simulink model "B1P3_Torsonal_Model_1_Coupler"  (Simulink 6.5)
settings: Solver=ode23tb  StartTime=0.0  StopTime=0.5  RelTol=1e-3
values from neighbouring files (symbols this model uses):
  B1 = 0    [B1P3_Torsonal_Model_1_Coupler_Constants.m]    (also in B1P6_Torsonal_Model_2_Coupler_Constants.m; Torsonal_Model_Constants.m)
  Bc = 0.01    [B1P3_Torsonal_Model_1_Coupler_Constants.m]    (also in Torsonal_Model_Constants.m)
  BL = 0    [B1P3_Torsonal_Model_1_Coupler_Constants.m]    (also in Torsonal_Model_Constants.m)
  J1 = 0.0033    [B1P3_Torsonal_Model_1_Coupler_Constants.m]    (also in B1P6_Torsonal_Model_2_Coupler_Constants.m = 0.0023; Torsonal_Model_Constants.m = 0.0023)
  JL = 0.0033    [B1P15_Torsonal_Model_From_V_Rizzo_One_Coupler_Constants.m]    (also in B1P3_Torsonal_Model_1_Coupler_Constants.m = 0.0023; RizzoConst.m; Torsonal_Model_Constants.m)
  K = 1000    [B1P3_Torsonal_Model_1_Coupler_Constants.m]    (also in Torsonal_Model_Constants.m = 55)
settings Model: Creator=dml46  LastModifiedBy=dml46

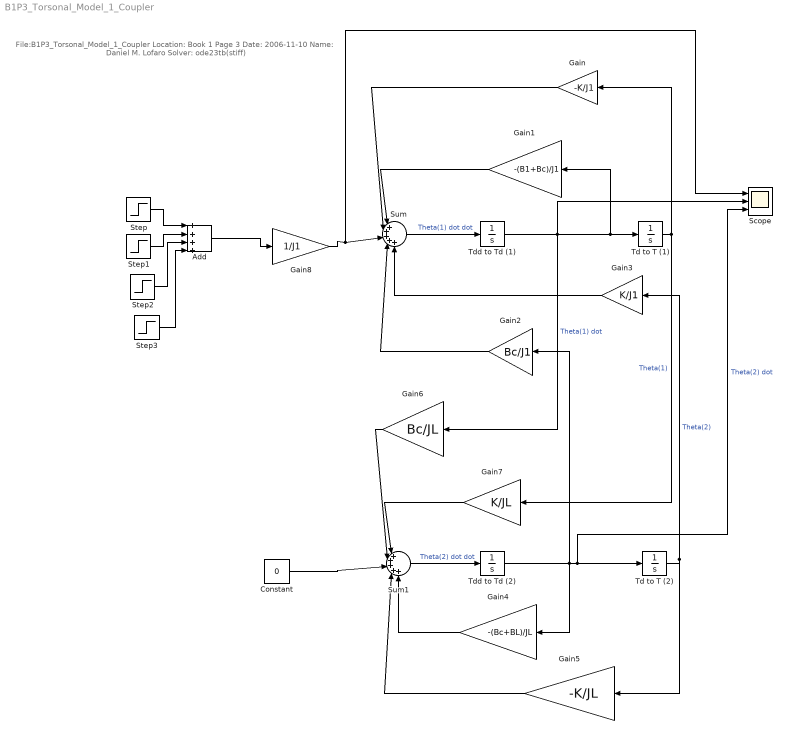
== system B1P3_Torsonal_Model_1_Coupler ==
  note: File:B1P3_Torsonal_Model_1_Coupler
      | Location: Book 1 Page 3
      | Date: 2006-11-10
      | Name: Daniel M. Lofaro
      | Solver: ode23tb(stiff)
  Add : Sum  Inputs=++++  OutScaling=2^-10
  Constant : Constant  Value=0  OutDataType=sfix(16)  ConRadixGroup=Use specified scaling  OutScaling=2^0  SampleTime=inf  FramePeriod=inf
  Gain : Gain  Orientation=left  Gain=-K/J1
  Gain1 : Gain  Orientation=left  Gain=-(B1+Bc)/J1
  Gain2 : Gain  Orientation=left  Gain=Bc/J1
  Gain3 : Gain  Orientation=left  Gain=K/J1
  Gain4 : Gain  Orientation=left  Gain=-(Bc+BL)/JL
  Gain5 : Gain  Orientation=left  Gain=-K/JL
  Gain6 : Gain  Orientation=left  Gain=Bc/JL
  Gain7 : Gain  Orientation=left  Gain=K/JL
  Gain8 : Gain  Gain=1/J1
  Scope : Scope  NumInputPorts=3
      settings: YMin=-5~-5~-5  YMax=5~5~5  MaxDataPoints=50000
  Step : Step  Time=0.1  SampleTime=0
  Step1 : Step  Time=0.2  After=-1  SampleTime=0
  Step2 : Step  Time=0.3  After=-1  SampleTime=0
  Step3 : Step  Time=0.4  SampleTime=0
  Sum : Sum  Inputs=|+++++
  Sum1 : Sum  Inputs=|+++++
  Td to T (1) : Integrator
  Td to T (2) : Integrator
  Tdd to Td (1) : Integrator
  Tdd to Td (2) : Integrator
  wires:
  Tdd to Td (2)/1 -> Gain2/1, Gain4/1, Td to T (2)/1, Scope/3  "Theta(2) dot"
  Tdd to Td (1)/1 -> Gain6/1, Td to T (1)/1, Gain1/1, Scope/2  "Theta(1) dot"
  Td to T (1)/1 -> Gain7/1, Gain/1  "Theta(1)"
  Sum/1 -> Tdd to Td (1)/1  "Theta(1) dot dot"
  Gain/1 -> Sum/2
  Gain1/1 -> Sum/1
  Sum1/1 -> Tdd to Td (2)/1  "Theta(2) dot dot"
  Gain2/1 -> Sum/4
  Gain3/1 -> Sum/5
  Td to T (2)/1 -> Gain5/1, Gain3/1  "Theta(2)"
  Gain4/1 -> Sum1/5
  Gain5/1 -> Sum1/4
  Gain6/1 -> Sum1/2
  Gain7/1 -> Sum1/1
  Constant/1 -> Sum1/3
  Step/1 -> Add/1
  Step1/1 -> Add/2
  Step2/1 -> Add/3
  Step3/1 -> Add/4
  Add/1 -> Gain8/1
  Gain8/1 -> Sum/3, Scope/1
